simulink model "angularacc"  (R2020a)
settings: Solver=VariableStepAuto  StartTime=0.0  StopTime=10.0  RelTol=1e-3
undefined symbols (not defined in the file): I, Ixx, Iyy, Izz, Jr
settings Model: Creator=Muni Kumar  LastModifiedBy=Muni Kumar

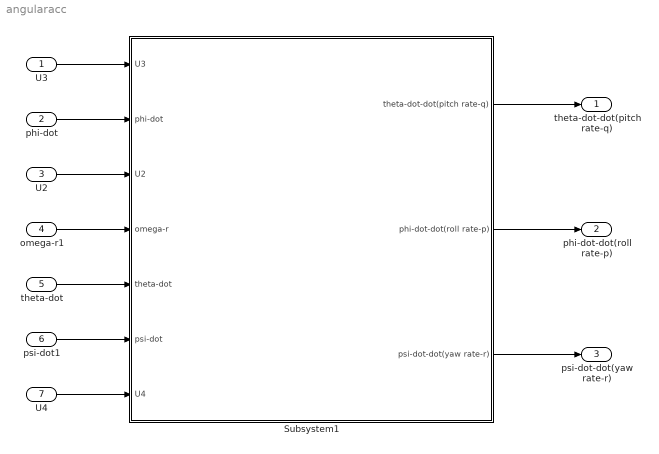
== system angularacc ==
  U3 : Inport
  phi-dot : Inport  Port=2
  U2 : Inport  Port=3
  omega-r1 : Inport  Port=4
  theta-dot : Inport  Port=5
  psi-dot1 : Inport  Port=6
  U4 : Inport  Port=7
  Subsystem1 : Subsystem
  theta-dot-dot(pitch rate-q) : Outport
  phi-dot-dot(roll rate-p) : Outport  Port=2
  psi-dot-dot(yaw rate-r) : Outport  Port=3
  wires:
  U3/1 -> Subsystem1/1(U3)
  phi-dot/1 -> Subsystem1/2(phi-dot)
  U2/1 -> Subsystem1/3(U2)
  omega-r1/1 -> Subsystem1/4(omega-r)
  theta-dot/1 -> Subsystem1/5(theta-dot)
  psi-dot1/1 -> Subsystem1/6(psi-dot)
  U4/1 -> Subsystem1/7(U4)
  Subsystem1/1(theta-dot-dot(pitch rate-q)) -> theta-dot-dot(pitch rate-q)/1
  Subsystem1/2(phi-dot-dot(roll rate-p)) -> phi-dot-dot(roll rate-p)/1
  Subsystem1/3(psi-dot-dot(yaw rate-r)) -> psi-dot-dot(yaw rate-r)/1

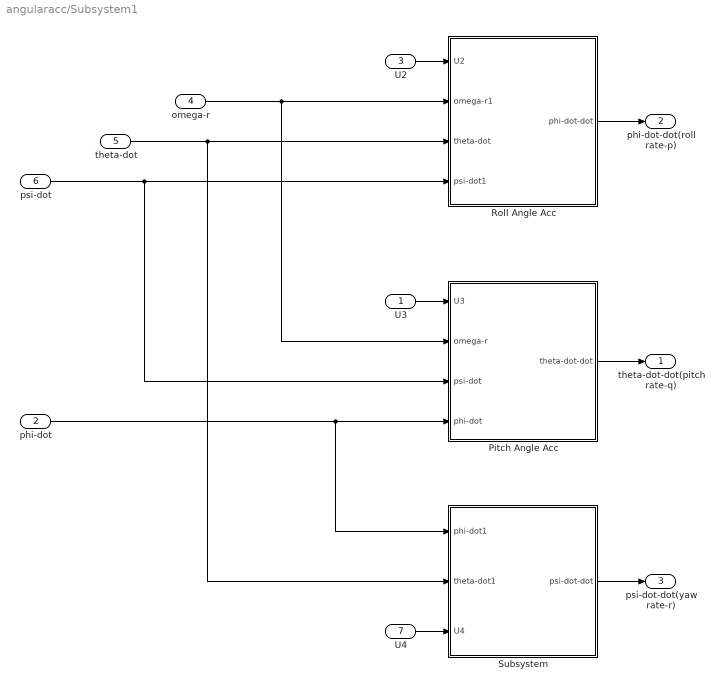
== system angularacc/Subsystem1 ==
  U3 : Inport
  phi-dot : Inport  Port=2
  U2 : Inport  Port=3
  omega-r : Inport  Port=4
  theta-dot : Inport  Port=5
  psi-dot : Inport  Port=6
  U4 : Inport  Port=7
  Pitch Angle Acc : Subsystem
  Roll Angle Acc : Subsystem
  Subsystem : Subsystem
  theta-dot-dot(pitch rate-q) : Outport
  phi-dot-dot(roll rate-p) : Outport  Port=2
  psi-dot-dot(yaw rate-r) : Outport  Port=3
  wires:
  phi-dot/1 -> Subsystem/1(phi-dot1), Pitch Angle Acc/4(phi-dot)
  U2/1 -> Roll Angle Acc/1(U2)
  Roll Angle Acc/1(phi-dot-dot) -> phi-dot-dot(roll rate-p)/1
  U4/1 -> Subsystem/3(U4)
  theta-dot/1 -> Subsystem/2(theta-dot1), Roll Angle Acc/3(theta-dot)
  Subsystem/1(psi-dot-dot) -> psi-dot-dot(yaw rate-r)/1
  psi-dot/1 -> Pitch Angle Acc/3(psi-dot), Roll Angle Acc/4(psi-dot1)
  Pitch Angle Acc/1(theta-dot-dot) -> theta-dot-dot(pitch rate-q)/1
  U3/1 -> Pitch Angle Acc/1(U3)
  omega-r/1 -> Pitch Angle Acc/2(omega-r), Roll Angle Acc/2(omega-r1)

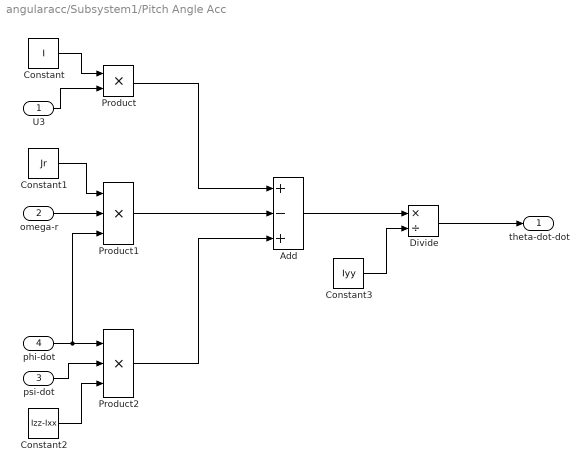
== system angularacc/Subsystem1/Pitch Angle Acc ==
  U3 : Inport
  omega-r : Inport  Port=2
  psi-dot : Inport  Port=3
  phi-dot : Inport  Port=4
  Add : Sum  Inputs=+-+
  Constant : Constant  Value=I
  Constant1 : Constant  Value=Jr
  Constant2 : Constant  Value=Izz-Ixx
  Constant3 : Constant  Value=Iyy
  Divide : Product  Inputs=*/
  Product : Product
  Product1 : Product  Inputs=3
  Product2 : Product  Inputs=3
  theta-dot-dot : Outport
  wires:
  Divide/1 -> theta-dot-dot/1
  Product/1 -> Add/1
  phi-dot/1 -> Product1/3, Product2/1
  psi-dot/1 -> Product2/2
  Product1/1 -> Add/2
  Constant1/1 -> Product1/1
  U3/1 -> Product/2
  Constant/1 -> Product/1
  Constant3/1 -> Divide/2
  Constant2/1 -> Product2/3
  omega-r/1 -> Product1/2
  Add/1 -> Divide/1
  Product2/1 -> Add/3

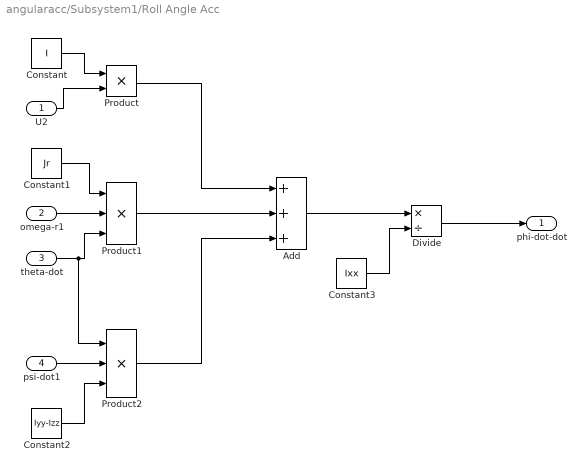
== system angularacc/Subsystem1/Roll Angle Acc ==
  U2 : Inport
  omega-r1 : Inport  Port=2
  theta-dot : Inport  Port=3
  psi-dot1 : Inport  Port=4
  Add : Sum  Inputs=+++
  Constant : Constant  Value=I
  Constant1 : Constant  Value=Jr
  Constant2 : Constant  Value=Iyy-Izz
  Constant3 : Constant  Value=Ixx
  Divide : Product  Inputs=*/
  Product : Product
  Product1 : Product  Inputs=3
  Product2 : Product  Inputs=3
  phi-dot-dot : Outport
  wires:
  psi-dot1/1 -> Product2/2
  Product/1 -> Add/1
  Constant/1 -> Product/1
  theta-dot/1 -> Product2/1, Product1/3
  Product1/1 -> Add/2
  Constant3/1 -> Divide/2
  Add/1 -> Divide/1
  Constant2/1 -> Product2/3
  Product2/1 -> Add/3
  U2/1 -> Product/2
  omega-r1/1 -> Product1/2
  Constant1/1 -> Product1/1
  Divide/1 -> phi-dot-dot/1

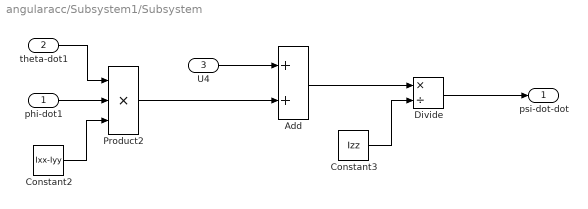
== system angularacc/Subsystem1/Subsystem ==
  phi-dot1 : Inport
  theta-dot1 : Inport  Port=2
  U4 : Inport  Port=3
  Add : Sum
  Constant2 : Constant  Value=Ixx-Iyy
  Constant3 : Constant  Value=Izz
  Divide : Product  Inputs=*/
  Product2 : Product  Inputs=3
  psi-dot-dot : Outport
  wires:
  Constant2/1 -> Product2/3
  phi-dot1/1 -> Product2/2
  Product2/1 -> Add/2
  theta-dot1/1 -> Product2/1
  Constant3/1 -> Divide/2
  Add/1 -> Divide/1
  U4/1 -> Add/1
  Divide/1 -> psi-dot-dot/1
